simulink model "rightLC"  (Simulink 7.7)
settings: Solver=ode45  StartTime=0.0  StopTime=1000  FixedStep=0.2  RelTol=1e-3
settings Model: Creator=jiannianweng  LastModifiedBy=jiannianweng

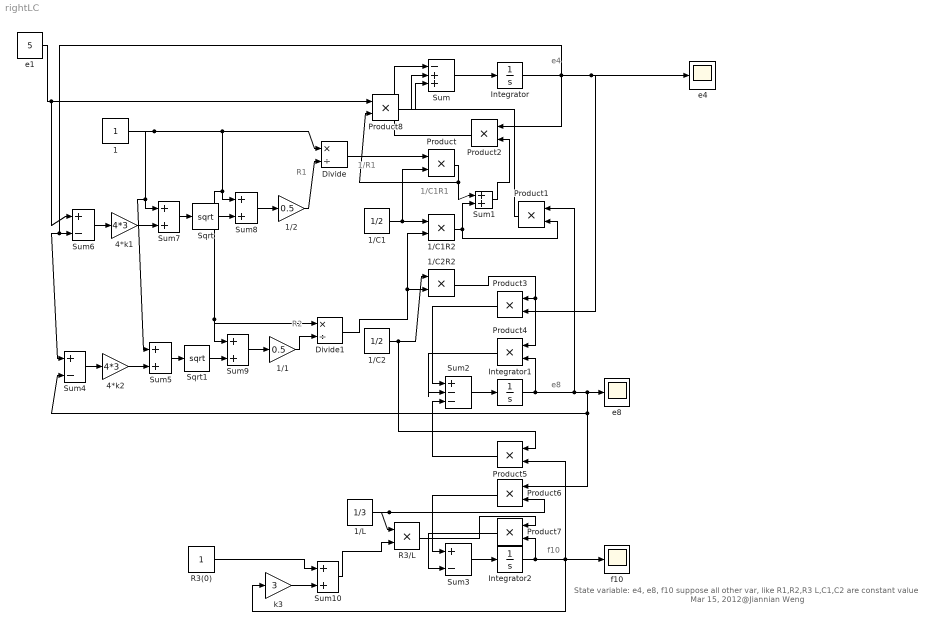
== system rightLC ==
  note: e4
  note: e8
  note: f10
  note: 1/C1R1
  note: State variable: e4, e8, f10
      | suppose all other var, like R1,R2,R3
      | L,C1,C2 are constant value
      | Mar 15, 2012@Jiannian Weng
  note: R1
  note: 1/R1
  note: R2
  1 : Constant
  1/1 : Gain  Gain=0.5
  1/2 : Gain  Gain=0.5
  1/C1 : Constant  Value=1/2
  1/C1R2 : Product  RndMeth=Zero
  1/C2 : Constant  Value=1/2
  1/C2R2 : Product  RndMeth=Zero
  1/L : Constant  Value=1/3
  4*k1 : Gain  Gain=4*3
  4*k2 : Gain  Gain=4*3
  Divide : Product  Inputs=*/
  Divide1 : Product  Inputs=*/
  Integrator : Integrator
  Integrator1 : Integrator
  Integrator2 : Integrator
  Product{,1..8} (9 alike) : Product  RndMeth=Zero
  R3(0) : Constant
  R3/L : Product  RndMeth=Zero
  Sqrt : Sqrt  OutputSignalType=real  SaturateOnIntegerOverflow=on
  Sqrt1 : Sqrt  OutputSignalType=real  SaturateOnIntegerOverflow=on
  Sum : Sum  Inputs=|-++
  Sum{1,5,7..10} (6 alike) : Sum  Inputs=|++
  Sum2 : Sum  Inputs=|+--
  Sum3 : Sum  Inputs=|+-
  Sum4 : Sum  Inputs=|+-
  Sum6 : Sum  Inputs=|+-
  e1 : Constant  Value=5
  e4 : Scope
      settings: YMin=2.49475  YMax=2.4995
  e8 : Scope
      settings: YMin=5.05e-06  YMax=5.85e-06
  f10 : Scope
      settings: YMin=4.99975e-06  YMax=4.99998e-06  SaveName=ScopeData2
  k3 : Gain  Gain=3
  wires:
  Integrator/1 -> Product2/1, e4/1, Product3/2, Sum6/2, Sum4/1
  Integrator1/1 -> Product1/1, e8/1, Product6/1, Sum4/2, Product4/2
  Integrator2/1 -> f10/1, Product5/2, k3/1, Product7/2
  Sum/1 -> Integrator/1
  1/C1/1 -> Product/2, 1/C1R2/1
  Product/1 -> Sum1/1, Product8/2
  1/C1R2/1 -> Sum1/2, Product1/2
  Sum1/1 -> Product2/2
  Product2/1 -> Sum/1
  Product1/1 -> Sum/2
  1/C2/1 -> 1/C2R2/1, Product5/1
  1/C2R2/1 -> Product3/1, Product4/1
  Sum2/1 -> Integrator1/1
  Product3/1 -> Sum2/1
  Product4/1 -> Sum2/2
  Product5/1 -> Sum2/3
  Sum3/1 -> Integrator2/1
  1/L/1 -> Product6/2, R3/L/1
  Product6/1 -> Sum3/1
  Sum10/1 -> R3/L/2
  R3/L/1 -> Product7/1
  Product7/1 -> Sum3/2
  Divide/1 -> Product/1
  1/1 -> Divide/1, Sum8/1, Sum9/1, Divide1/1, Sum7/1, Sum5/1
  e1/1 -> Product8/1, Sum6/1
  Product8/1 -> Sum/3
  Sum6/1 -> 4*k1/1
  4*k1/1 -> Sum7/2
  Sum7/1 -> Sqrt/1
  Sqrt/1 -> Sum8/2
  Sum8/1 -> 1/2/1
  1/2/1 -> Divide/2
  Sum4/1 -> 4*k2/1
  4*k2/1 -> Sum5/2
  Sum5/1 -> Sqrt1/1
  Sqrt1/1 -> Sum9/2
  Sum9/1 -> 1/1/1
  1/1/1 -> Divide1/2
  Divide1/1 -> 1/C1R2/2, 1/C2R2/2
  k3/1 -> Sum10/2
  R3(0)/1 -> Sum10/1
